simulink model "WindFarmGFMControlFast"  (R2023a)
settings: Solver=VariableStepAuto  StartTime=0.0  StopTime=Tsim  FixedStep=Ts  MaxStep=1  MinStep=Ts  RelTol=1e-3
PreLoadFcn:
  | run('WindFarmGFMControlParametersFast.m')
undefined symbols (not defined in the file): DiscIntNeverNeededParam, feeder, frt, gGFM, grid, line, loads, lvrt, mGFM, pmsm, time, Ts, windController, windTransformer, windTurbine
libraries: ee_lib x21, nesl_utility x14, eeGeneralControl x4, fl_lib x3, spsLeadLagFilterLib x2, eeTransforms x2, eePowerMeasurement x1, eeSinusoidalMeasurementV2 x1
(part 2 of 2)

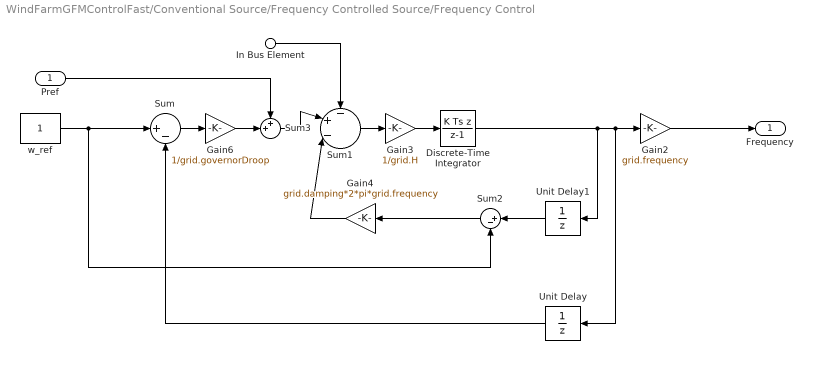
== system WindFarmGFMControlFast/Conventional Source/Frequency Controlled Source/Frequency Control ==
  Pref : Inport
  In Bus Element : Inport  Port=2  PortName=Grid  Element=Pe
  Discrete-Time Integrator : DiscreteIntegrator  IntegratorMethod=Integration: Backward Euler  InitialCondition=1  SampleTime=Ts  LimitOutput=on  UpperSaturationLimit=1.1  LowerSaturationLimit=0.9  ICPrevOutput=DiscIntNeverNeededParam  ICPrevScaledInput=DiscIntNeverNeededParam
  Gain2 : Gain  Gain=grid.frequency
  Gain3 : Gain  Gain=1/grid.H
  Gain4 : Gain  Gain=grid.damping*2*pi*grid.frequency
  Gain6 : Gain  Gain=1/grid.governorDroop
  Sum : Sum  Inputs=|+-
  Sum1 : Sum  Inputs=-+-|
  Sum2 : Sum  Inputs=|+-
  Sum3 : Sum  Inputs=++|
  Unit Delay : UnitDelay  InitialCondition=1  SampleTime=grid.sensorTime  HasFrameUpgradeWarning=on
  Unit Delay1 : UnitDelay  InitialCondition=1  SampleTime=grid.sensorTime  HasFrameUpgradeWarning=on
  w_ref : Constant
  Frequency : Outport
  wires:
  Sum3/1 -> Sum1/2
  w_ref/1 -> Sum2/2, Sum/1
  Sum1/1 -> Gain3/1
  Gain3/1 -> Discrete-Time Integrator/1
  Gain6/1 -> Sum3/2
  Gain2/1 -> Frequency/1
  Sum2/1 -> Gain4/1
  Sum/1 -> Gain6/1
  Pref/1 -> Sum3/1
  Gain4/1 -> Sum1/3
  In Bus Element/1 -> Sum1/1
  Discrete-Time Integrator/1 -> Unit Delay1/1, Unit Delay/1, Gain2/1
  Unit Delay/1 -> Sum/2
  Unit Delay1/1 -> Sum2/1

== system WindFarmGFMControlFast/Wind Farm/Voltage VAR Control & LVRT, FRT/Frequency RideThrough ==
  f : Inport
  Avoid Operation : Subsystem
  Discrete-Time Integrator1 : DiscreteIntegrator  ExternalReset=either  SampleTime=Ts  ICPrevOutput=DiscIntNeverNeededParam  ICPrevScaledInput=DiscIntNeverNeededParam
  Duration of f<fth : Lookup_n-D  NumberOfTableDimensions=1  BreakpointsForDimension1=(1+[-0.021,-0.02,0.02,0.021])*grid.frequency  Table=[1,0,0,1]  InterpMethod=Flat  InternalRulePriority=Speed  RndMeth=Simplest
  Frequency vs Trip time : Lookup_n-D  NumberOfTableDimensions=1  BreakpointsForDimension1=frt.frequency  Table=frt.time  InterpMethod=Flat  InternalRulePriority=Speed  RndMeth=Simplest
  GreaterThan : RelationalOperator  Operator=>  OutDataTypeStr=boolean  RndMeth=Simplest  InputSameDT=off
  Trip  Signal : Outport
  wires:
  Discrete-Time Integrator1/1 -> GreaterThan/1
  Frequency vs Trip time/1 -> GreaterThan/2
  GreaterThan/1 -> Trip  Signal/1
  Duration of f<fth/1 -> Discrete-Time Integrator1/2, Discrete-Time Integrator1/1
  Avoid Operation/1(f) -> Duration of f<fth/1, Frequency vs Trip time/1
  f/1 -> Avoid Operation/1(f_in)

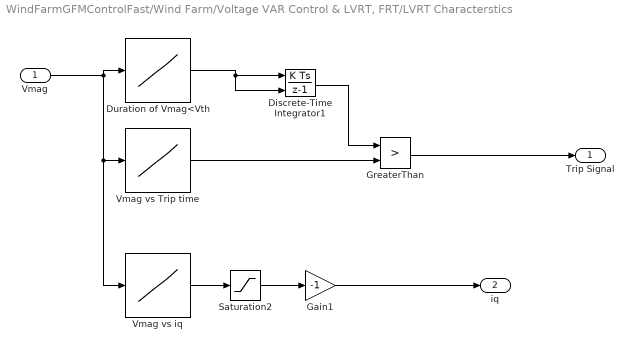
== system WindFarmGFMControlFast/Wind Farm/Voltage VAR Control & LVRT, FRT/LVRT Characterstics ==
  Vmag : Inport
  Discrete-Time Integrator1 : DiscreteIntegrator  ExternalReset=either  SampleTime=Ts  ICPrevOutput=DiscIntNeverNeededParam  ICPrevScaledInput=DiscIntNeverNeededParam
  Duration of Vmag<Vth : Lookup_n-D  NumberOfTableDimensions=1  BreakpointsForDimension1=[0,.9,0.91,1.2]  Table=[1,1,0,0]  InterpMethod=Flat  InternalRulePriority=Speed  RndMeth=Simplest
  Gain1 : Gain  Gain=-1
  GreaterThan : RelationalOperator  Operator=>  OutDataTypeStr=boolean  RndMeth=Simplest  InputSameDT=off
  Saturation2 : Saturate  UpperLimit=1/8  LowerLimit=-1
  Vmag vs Trip time : Lookup_n-D  NumberOfTableDimensions=1  BreakpointsForDimension1=lvrt.voltage  Table=lvrt.time  InterpMethod=Flat  InternalRulePriority=Speed  RndMeth=Simplest
  Vmag vs iq : Lookup_n-D  NumberOfTableDimensions=1  BreakpointsForDimension1=lvrt.voltageiq  Table=lvrt.iq  InternalRulePriority=Speed  RndMeth=Simplest
  Trip Signal : Outport
  iq : Outport  Port=2
  wires:
  Duration of Vmag<Vth/1 -> Discrete-Time Integrator1/2, Discrete-Time Integrator1/1
  GreaterThan/1 -> Trip Signal/1
  Discrete-Time Integrator1/1 -> GreaterThan/1
  Vmag vs Trip time/1 -> GreaterThan/2
  Vmag vs iq/1 -> Saturation2/1
  Gain1/1 -> iq/1
  Saturation2/1 -> Gain1/1
  Vmag/1 -> Vmag vs iq/1, Vmag vs Trip time/1, Duration of Vmag<Vth/1

== system WindFarmGFMControlFast/Wind Farm/Voltage VAR Control & LVRT, FRT/Voltage Control ==
  In1 : Inport
  In2 : Inport  Port=2
  Constant2 : Constant  Value=0
  Gain : Gain  Gain=windController.mv
  Sum2 : Sum  Inputs=|+-
  Switch1 : Switch  Threshold=.9  SaturateOnIntegerOverflow=off  InputSameDT=off
  Out1 : Outport
  wires:
  Gain/1 -> Out1/1
  Sum2/1 -> Switch1/1
  Switch1/1 -> Gain/1
  In1/1 -> Sum2/2, Switch1/2
  Constant2/1 -> Switch1/3
  In2/1 -> Sum2/1

== system WindFarmGFMControlFast/Wind Farm/Voltage VAR Control & LVRT, FRT/Frequency RideThrough/Avoid Operation ==
  f_in : Inport
  Constant : Constant  Value=grid.frequency  SampleTime=Ts
  Step : Step  Time=0.5  SampleTime=Ts
  Switch : Switch  Criteria=u2 > Threshold  SaturateOnIntegerOverflow=off  InputSameDT=off
  f : Outport
  wires:
  f_in/1 -> Switch/1
  Constant/1 -> Switch/3
  Step/1 -> Switch/2
  Switch/1 -> f/1
